simulink model "assignment_7_pd_invdyn"  (R2022b)
settings: Solver=VariableStepAuto  StartTime=0.0  StopTime=10.0  RelTol=1e-3
values from neighbouring files (symbols this model uses):
  dq0 = [0;0;0]    [assignment_10.m]    (also in assignment_11.m; assignment_12.m; assignment_13.m; assignment_6.m)
  Kd = 100    [assignment_10.m]    (also in assignment_11.m = 1000; assignment_12.m; assignment_6.m = 1000; assignment_7.m = diag(2 * xi .* w))
  Kp = 1000    [assignment_10.m]    (also in assignment_11.m = 10000; assignment_12.m; assignment_6.m; assignment_7.m = diag(w .* w))
  q0 = [0;0;0]    [assignment_10.m]    (also in assignment_11.m; assignment_12.m; assignment_13.m = [0; pi/2; -pi/2]; assignment_6.m)
  traj = [q1_d; q2_d; q3_d]    [assignment_10.m]    (also in assignment_12.m; assignment_7.m)
undefined symbols (not defined in the file or in its folder): sigbuilder_block
libraries: robotcorelib x1
settings Model: Creator=acesi  LastModifiedBy=Manu

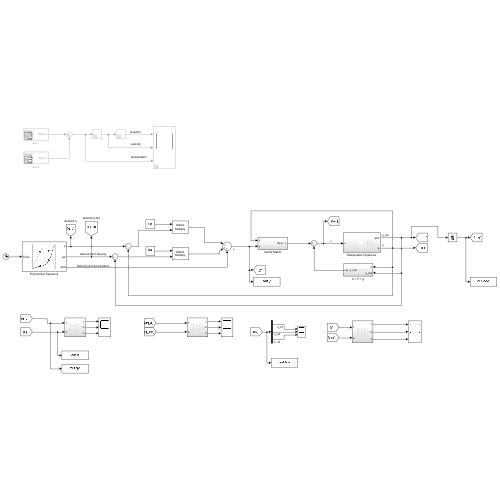
[thumbnail: Simulink's stored preview of the top-level diagram]
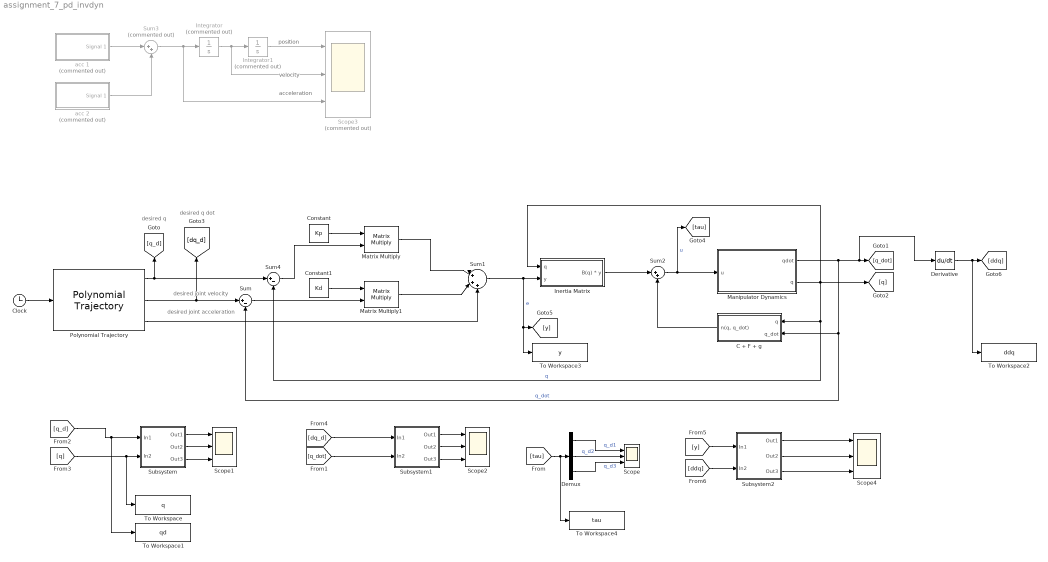
== system assignment_7_pd_invdyn ==
  note: desired q
  note: position
  note: velocity
  note: acceleration
  note: desired joint velocity
  note: desired joint acceleration
  note: desired q dot
  C + F + g : Subsystem
  Clock : Clock
  Constant : Constant  Value=Kp
  Constant1 : Constant  Value=Kd
  Demux : Demux  Outputs=3
  Derivative : Derivative
  Inertia Matrix : Subsystem
  Integrator : Integrator  Commented=on
  Integrator1 : Integrator  Commented=on
  Manipulator Dynamics : Subsystem
  Matrix Multiply : Product  Multiplication=Matrix(*)
  Matrix Multiply1 : Product  Multiplication=Matrix(*)
  Polynomial Trajectory : robotcorelib/Polynomial Trajectory  WaypointSource=Internal  Waypoints=traj  TimePoints=time_vector  TimeInterval=[ 1, 4 ]  Method=Quintic Polynomial  ParameterSource=Internal  VelocityBoundaryCondition=zeros(size(traj))  AccelerationBoundaryCondition=zeros(size(traj))  SimulateUsing=Interpreted execution
  Scope{,1..2,4} (4 alike) : Scope  NumInputPorts=3
  Scope3 : Scope  Commented=on  NumInputPorts=3
  Subsystem : Subsystem
  Subsystem1 : Subsystem
  Subsystem2 : Subsystem
  Sum : Sum  Inputs=|+-
  Sum1 : Sum  Inputs=|+++
  Sum2 : Sum  Inputs=|++
  Sum3 : Sum  Commented=on  Inputs=|++
  Sum4 : Sum  Inputs=|+-
  To Workspace : ToWorkspace  VariableName=q  SaveFormat=Timeseries  SampleTime=-1
  To Workspace1 : ToWorkspace  VariableName=qd  SaveFormat=Timeseries  SampleTime=-1
  To Workspace2 : ToWorkspace  VariableName=ddq  SaveFormat=Timeseries  SampleTime=-1
  To Workspace3 : ToWorkspace  VariableName=y  SaveFormat=Timeseries  SampleTime=-1
  To Workspace4 : ToWorkspace  VariableName=tau  SaveFormat=Timeseries  SampleTime=-1
  acc 1 : Subsystem  Tag=STV Subsys  Commented=on  LoadFcn=sigbuilder_block('load');  StartFcn=sigbuilder_block('start');  StopFcn=sigbuilder_block('stop');  ClipboardFcn=sigbuilder_block('clipboard');  mask(Sigbuilder block){tuvar=[0:10]}
      mask help: Simulink:masks:SigbuilderBlock_MD
      mask init:
      | if ~strcmp(get_param(bdroot(gcbh),'SimulationStatus'),'stopped') tuvar = sigbuilder_block('maskInit'); end
      settings: CopyFcn=sigbuilder_block('copy');  DeleteFcn=sigbuilder_block('delete');  ModelCloseFcn=sigbuilder_block('modelClose');  PreSaveFcn=sigbuilder_block('preSave');  PauseFcn=sigbuilder_block('pause');  ContinueFcn=sigbuilder_block('continue');  NameChangeFcn=sigbuilder_block('namechange');  OpenFcn=sigbuilder_block('open',[437.6 199.2 550.4 400 ]);  CloseFcn=sigbuilder_block('close');
      mask Display: plot(0, 0, 100, 100,[2, 2, 32, 32, 2], [68, 8, 8, 68, 68],[32, 2], [38, 38], [32, 19, 2],[53, 60, 44], [32, 17, 17, 2],[16, 16, 31, 31]);txt = getActiveGroup(gcbh);text(2, 100, txt,'verticalAlignment', 'top');
  acc 2 : Subsystem  Tag=STV Subsys  Commented=on  LoadFcn=sigbuilder_block('load');  StartFcn=sigbuilder_block('start');  StopFcn=sigbuilder_block('stop');  ClipboardFcn=sigbuilder_block('clipboard');  mask(Sigbuilder block){tuvar=[0:10]}
      mask help: Simulink:masks:SigbuilderBlock_MD
      mask init:
      | if ~strcmp(get_param(bdroot(gcbh),'SimulationStatus'),'stopped') tuvar = sigbuilder_block('maskInit'); end
      settings: CopyFcn=sigbuilder_block('copy');  DeleteFcn=sigbuilder_block('delete');  ModelCloseFcn=sigbuilder_block('modelClose');  PreSaveFcn=sigbuilder_block('preSave');  PauseFcn=sigbuilder_block('pause');  ContinueFcn=sigbuilder_block('continue');  NameChangeFcn=sigbuilder_block('namechange');  OpenFcn=sigbuilder_block('open',[403.5 84.75 550.5 363.75 ]);  CloseFcn=sigbuilder_block('close');
      mask Display: plot(0, 0, 100, 100,[2, 2, 32, 32, 2], [68, 8, 8, 68, 68],[32, 2], [38, 38], [32, 19, 2],[53, 60, 44], [32, 17, 17, 2],[16, 16, 31, 31]);txt = getActiveGroup(gcbh);text(2, 100, txt,'verticalAlignment', 'top');
  wires:
  Manipulator Dynamics/1(qdot) -> Derivative/1, [q_dot], C + F + g/2(q_dot), Sum/2  "q_dot"
  Manipulator Dynamics/2(q) -> Sum4/2, C + F + g/1(q), [q], Inertia Matrix/1(q)  "q"
  Inertia Matrix/1(B(q) * y) -> Sum2/1
  Sum2/1 -> [tau], Manipulator Dynamics/1(u)  "u"
  C + F + g/1("n(q, q_dot)") -> Sum2/2
  Polynomial Trajectory/1 -> [q_d], Sum4/1
  [q_d] -> Subsystem/1(In1), To Workspace1/1
  [q] -> To Workspace/1, Subsystem/2(In2)
  Subsystem/1(Out1) -> Scope1/1
  Subsystem/2(Out2) -> Scope1/2
  Subsystem/3(Out3) -> Scope1/3
  [dq_d] -> Subsystem1/1(In1)
  [q_dot] -> Subsystem1/2(In2)
  Subsystem1/1(Out1) -> Scope2/1
  Subsystem1/2(Out2) -> Scope2/2
  Subsystem1/3(Out3) -> Scope2/3
  acc 1/1(Signal 1) -> Sum3/1
  acc 2/1(Signal 1) -> Sum3/2
  Sum3/1 -> Scope3/3, Integrator/1
  Integrator/1 -> Scope3/2, Integrator1/1
  Integrator1/1 -> Scope3/1
  Clock/1 -> Polynomial Trajectory/1
  Polynomial Trajectory/3 -> Sum1/3
  Polynomial Trajectory/2 -> Sum/1, [dq_d]
  Matrix Multiply/1 -> Sum1/1
  Constant/1 -> Matrix Multiply/1
  Matrix Multiply1/1 -> Sum1/2
  Constant1/1 -> Matrix Multiply1/1
  Sum1/1 -> [y], To Workspace3/1, Inertia Matrix/2(y)  "e"
  Sum/1 -> Matrix Multiply1/2
  Sum4/1 -> Matrix Multiply/2
  Derivative/1 -> To Workspace2/1, [ddq]
  [y] -> Subsystem2/1(In1)
  [ddq] -> Subsystem2/2(In2)
  Subsystem2/1(Out1) -> Scope4/1
  Subsystem2/2(Out2) -> Scope4/2
  Subsystem2/3(Out3) -> Scope4/3
  [tau] -> To Workspace4/1, Demux/1
  Demux/1 -> Scope/1  "q_d1"
  Demux/2 -> Scope/2  "q_d2"
  Demux/3 -> Scope/3  "q_d3"

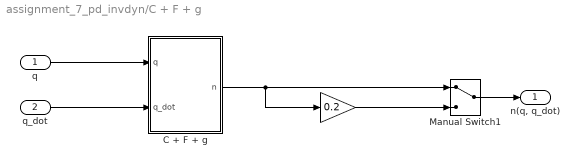
== system assignment_7_pd_invdyn/C + F + g ==
  q : Inport
  q_dot : Inport  Port=2
  " " : Gain  Gain=0.2
  C + F + g : MATLAB Function  TreatAsAtomicUnit=on
  Manual Switch1 : ManualSwitch
  "n(q, q_dot)" : Outport
  wires:
  q/1 -> C + F + g/1(q)
  q_dot/1 -> C + F + g/2(q_dot)
  C + F + g/1(n) -> " "/1, Manual Switch1/1
  " "/1 -> Manual Switch1/2
  Manual Switch1/1 -> "n(q, q_dot)"/1

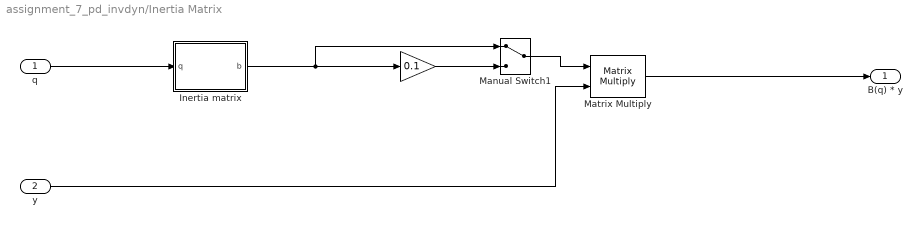
== system assignment_7_pd_invdyn/Inertia Matrix ==
  q : Inport
  y : Inport  Port=2
  " " : Gain  Gain=0.1
  Inertia matrix : MATLAB Function  TreatAsAtomicUnit=on
  Manual Switch1 : ManualSwitch
  Matrix Multiply : Product  Multiplication=Matrix(*)
  B(q) * y : Outport
  wires:
  q/1 -> Inertia matrix/1(q)
  y/1 -> Matrix Multiply/2
  Matrix Multiply/1 -> B(q) * y/1
  Inertia matrix/1(b) -> Manual Switch1/1, " "/1
  " "/1 -> Manual Switch1/2
  Manual Switch1/1 -> Matrix Multiply/1

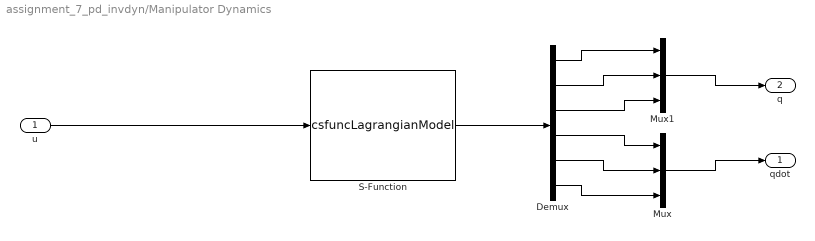
== system assignment_7_pd_invdyn/Manipulator Dynamics ==
  u : Inport
  Demux : Demux  Outputs=6
  Mux : Mux  Inputs=3
  Mux1 : Mux  Inputs=3
  S-Function : S-Function  FunctionName=csfuncLagrangianModel  Parameters=q0 dq0  SFunctionDeploymentMode=off  EnableBusSupport=off
  qdot : Outport
  q : Outport  Port=2
  wires:
  u/1 -> S-Function/1
  S-Function/1 -> Demux/1
  Mux1/1 -> q/1
  Mux/1 -> qdot/1
  Demux/6 -> Mux/3
  Demux/5 -> Mux/2
  Demux/4 -> Mux/1
  Demux/3 -> Mux1/3
  Demux/2 -> Mux1/2
  Demux/1 -> Mux1/1

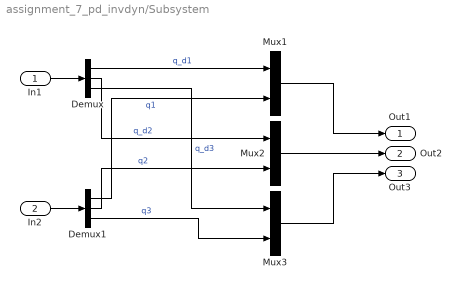
== system assignment_7_pd_invdyn/Subsystem ==
  In1 : Inport
  In2 : Inport  Port=2
  Demux : Demux  Outputs=3
  Demux1 : Demux  Outputs=3
  Mux1 : Mux  Inputs=2
  Mux2 : Mux  Inputs=2
  Mux3 : Mux  Inputs=2
  Out1 : Outport
  Out2 : Outport  Port=2
  Out3 : Outport  Port=3
  wires:
  Demux/1 -> Mux1/1  "q_d1"
  Demux/3 -> Mux3/1  "q_d3"
  Demux/2 -> Mux2/1  "q_d2"
  Demux1/1 -> Mux1/2  "q1"
  Mux2/1 -> Out2/1
  Demux1/3 -> Mux3/2  "q3"
  Demux1/2 -> Mux2/2  "q2"
  Mux3/1 -> Out3/1
  Mux1/1 -> Out1/1
  In2/1 -> Demux1/1
  In1/1 -> Demux/1

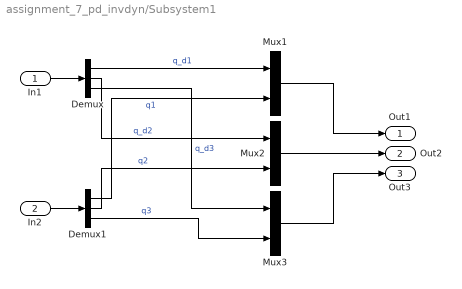
== system assignment_7_pd_invdyn/Subsystem1 ==
  In1 : Inport
  In2 : Inport  Port=2
  Demux : Demux  Outputs=3
  Demux1 : Demux  Outputs=3
  Mux1 : Mux  Inputs=2
  Mux2 : Mux  Inputs=2
  Mux3 : Mux  Inputs=2
  Out1 : Outport
  Out2 : Outport  Port=2
  Out3 : Outport  Port=3
  wires:
  Demux/1 -> Mux1/1  "q_d1"
  Demux/3 -> Mux3/1  "q_d3"
  Demux/2 -> Mux2/1  "q_d2"
  Demux1/1 -> Mux1/2  "q1"
  Mux2/1 -> Out2/1
  Demux1/3 -> Mux3/2  "q3"
  Demux1/2 -> Mux2/2  "q2"
  Mux3/1 -> Out3/1
  Mux1/1 -> Out1/1
  In2/1 -> Demux1/1
  In1/1 -> Demux/1

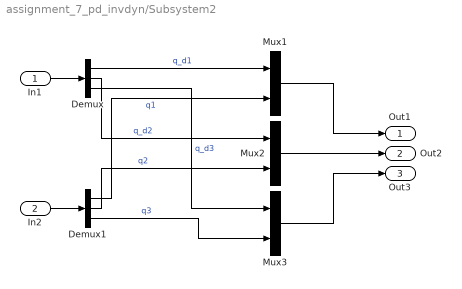
== system assignment_7_pd_invdyn/Subsystem2 ==
  In1 : Inport
  In2 : Inport  Port=2
  Demux : Demux  Outputs=3
  Demux1 : Demux  Outputs=3
  Mux1 : Mux  Inputs=2
  Mux2 : Mux  Inputs=2
  Mux3 : Mux  Inputs=2
  Out1 : Outport
  Out2 : Outport  Port=2
  Out3 : Outport  Port=3
  wires:
  Demux/1 -> Mux1/1  "q_d1"
  Demux/3 -> Mux3/1  "q_d3"
  Demux/2 -> Mux2/1  "q_d2"
  Demux1/1 -> Mux1/2  "q1"
  Mux2/1 -> Out2/1
  Demux1/3 -> Mux3/2  "q3"
  Demux1/2 -> Mux2/2  "q2"
  Mux3/1 -> Out3/1
  Mux1/1 -> Out1/1
  In2/1 -> Demux1/1
  In1/1 -> Demux/1

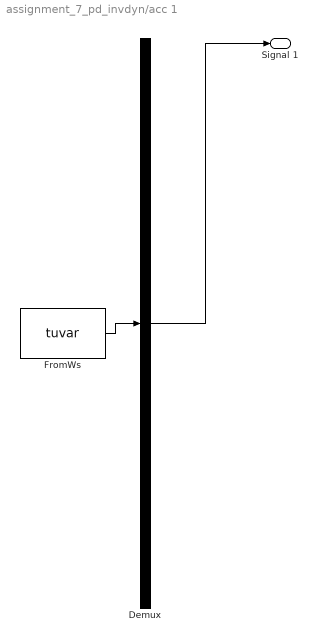
== system assignment_7_pd_invdyn/acc 1 ==
  Demux : Demux  Tag=STV Demux  Outputs=1
      settings: DisplayOption=none
  FromWs : FromWorkspace  Tag=STV FromWs  VariableName=tuvar
      SigBuilderData=|
      | common.afterFinalStr = 'Extrapolate'
      | common.sampleTime = 0
      | dataSet.timeRange = [0 10]
      | dataSet.name = 'Group 1'
      | sbobj.Groups.Name = 'Group 1'
      | sbobj.Groups.Signals.Name = 'Signal 1'
      | sbobj.Groups.Signals.XData = [0 1 1 3 3 10]
      | sbobj.Groups.Signals.YData = [0 0 1 1 0 0]
  Signal 1 : Outport  Tag=STV Outport
  wires:
  Demux/1 -> Signal 1/1
  FromWs/1 -> Demux/1

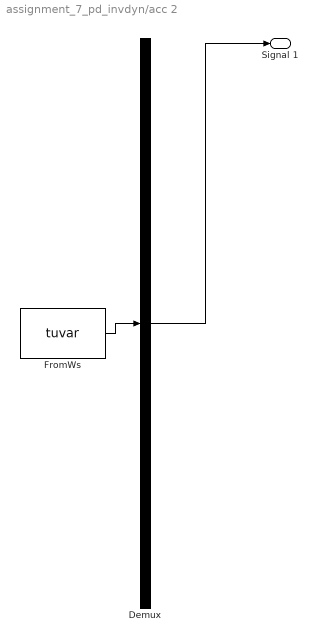
== system assignment_7_pd_invdyn/acc 2 ==
  Demux : Demux  Tag=STV Demux  Outputs=1
      settings: DisplayOption=none
  FromWs : FromWorkspace  Tag=STV FromWs  VariableName=tuvar
      SigBuilderData=|
      | common.afterFinalStr = 'Extrapolate'
      | common.sampleTime = 0
      | dataSet.timeRange = [0 10]
      | dataSet.name = 'Group 1'
      | sbobj.Groups.Name = 'Group 1'
      | sbobj.Groups.Signals.Name = 'Signal 1'
      | sbobj.Groups.Signals.XData = [0 6 6 9 9 10]
      | sbobj.Groups.Signals.YData = [0 0 -1 -1 0 0]
  Signal 1 : Outport  Tag=STV Outport
  wires:
  Demux/1 -> Signal 1/1
  FromWs/1 -> Demux/1

== matlab function assignment_7_pd_invdyn/C + F + g/C + F + g ==
  data: q input; n output; q_dot input
function n = N(q, q_dot)
    % return n = C(q, qd) + F + g(q) 

    g = get_G_hardcoded(q);
    c = get_C_hardcoded(q, q_dot) * q_dot;

    n = g + c;
end

== matlab function assignment_7_pd_invdyn/Inertia Matrix/Inertia matrix ==
  data: q input; b output
function b = B(q)

    b = get_B_hardcoded(q);

end
